simulink model "Tricopter_Controlled_development"  (R2015a)
settings: Solver=ode2  SolverMode=SingleTasking  StartTime=0.0  StopTime=inf  FixedStep=T_sim  RelTol=1e-3
values from neighbouring files (symbols this model uses):
  A_l_max_x = sqrt( (A_z_max)^2  -  g^2  )    [Run3Copter.m]
  A_l_max_y = g*tand(15)    [Run3Copter.m]
  A_x = 0.015    [SetupComplete.m]
  A_y = A_x    (= 0.015)    [SetupComplete.m]
  A_z = 0.16    [SetupComplete.m]
  A_z_max = Max_Thrust*3/m    [Run3Copter.m]
  Alt_0 = input(' Give the initial altitude (m): ')    [Run3Copter.m]
  C_x = 1.2    [SetupComplete.m]
  C_y = C_x    (= 1.2)    [SetupComplete.m]
  C_z = 2.2    [SetupComplete.m]
  CG_0 = [0,0,0.02]'    [SetupComplete.m]
  epsilon = 0.01    [Run3Copter.m]
  eta_23 = deg2rad(-1.3)    [Run3Copter.m]
  g = 9.81    [SetupComplete.m]
  h = 0.08    [SetupComplete.m]
  h_M = 0.064    [SetupComplete.m]
  I_BAC_0 = [ Ix,0,Ixz;0,Iy,0;Ixz,0,Iz]    [SetupComplete.m]
  Initial_Omegas = Omega_hover    [Run3Copter.m]
  Initial_Torques = Torque_hover    [Run3Copter.m]
  Ix = 0.103    [SetupComplete.m]
  Iy = 0.147    [SetupComplete.m]
  Iz = 0.237    [SetupComplete.m]
  l = 0.345    [SetupComplete.m]
  l_arm = 0.264    [SetupComplete.m]
  latitude = 52.071118    [Run3Copter.m]
  longitude = -0.627404    [Run3Copter.m]
  m = 3.51    [SetupComplete.m]
  m_0 = 2.61    [SetupComplete.m]
  m_M = 0.300    (= 0.3)    [SetupComplete.m]
  rho = 1.15    [SetupComplete.m]
  Rotation_sign = [ 1,-1,-1]    [SetupComplete.m]
  T_ctrl = 0.02    [Run3Copter.m]
  T_sim = 0.01    [Run3Copter.m]
  throtle_1 = 0*0.745    (= 0)    [Run3Copter.m]
  throtle_23 = throtle_1/cos(eta_23)    [Run3Copter.m]
  v_i0 = sqrt( 1/3*m*g/(2*rho*pi*R^2)  )    [SetupComplete.m]
undefined symbols (not defined in the file or in its folder): DOWN_0, EAST_0, Newton, NORTH_0, P_0, Q_0, R_0, Raphson, U_0, V_0, W_0
libraries: Adaptive_FaultTolerantControl x30, XXCopter_Control x23, simulink_extras x17, XXCopter x5, simulink x2, qcatlib x1, XXCopter_C x1
(part 4 of 4)

== matlab function Tricopter_Controlled_development/Parameters estimation/MATLAB Function ==
  data: T_yaw output; yaw input
function T_yaw = Yaw_rotate(yaw)


T_yaw=[cos(yaw),    sin(yaw),   0;
        -sin(yaw),  cos(yaw),   0;
        0,      0,              1];

== matlab function Tricopter_Controlled_development/3 Copter Complete/Ground  model/Ground model logic and Forces and moments ==
  data: Xe input; Vb input; q input; omega_b input; F_gr_b output; M_gr_b output; mass input; g parameter; Arm1 input; Arm2 input; Arm3 input
function [F_gr_b,M_gr_b]   = Gorund_Forces_and_Mom( Xe,Vb,q,omega_b,mass, g, Arm1,Arm2,Arm3)

F_gr_b=zeros(3,1);
M_gr_b=zeros(3,1);


% Arm 1
Prod=HamiltonProduct([q(1);q(2);q(3);q(4)],HamiltonProduct([0;Arm1],[q(1);-q(2);-q(3);-q(4)]) ); % q . Arm .q*: From body to earth axes
h_arm1 = Xe(3) + Prod(2:4);
% Arm 2
Prod=HamiltonProduct([q(1);q(2);q(3);q(4)],HamiltonProduct([0;Arm2],[q(1);-q(2);-q(3);-q(4)]) ); % q . Arm .q*: From body to earth axes
h_arm2 = Xe(3) + Prod(2:4);
% Arm 3
Prod=HamiltonProduct([q(1);q(2);q(3);q(4)],HamiltonProduct([0;Arm3],[q(1);-q(2);-q(3);-q(4)]) ); % q . Arm .q*: From body to earth axes
h_arm3 = Xe(3) + Prod(2:4);


min_h = max([Xe(3),h_arm1(3),h_arm2(3),h_arm3(3)]);
if min_h >=-0.01  &&  min_h <= 0  && Vb(3)>0
    Prod=HamiltonProduct([q(1);-q(2);-q(3);-q(4)],HamiltonProduct([0;0;0;-mass*g],[q(1);q(2);q(3);q(4)]) ); % q* . g .q: From earth to Body axes
    F_gr_b= Prod(2:4);
    %Friction forces
    F_gr_b = F_gr_b - 5*Vb;
    
elseif min_h >=-0.01  &&  min_h >0
    Prod=HamiltonProduct([q(1);-q(2);-q(3);-q(4)],HamiltonProduct([0;0;0; -5000*min_h ],[q(1);q(2);q(3);q(4)]) ); % q* . g .q: From earth to Body axes
    F_gr_b =  Prod(2:4);
    %Friction forces
    F_gr_b = F_gr_b - 250*Vb;
else
    F_gr_b=zeros(3,1);

end


% Moments
Prod=HamiltonProduct([q(1);-q(2);-q(3);-q(4)],HamiltonProduct([0;0;0;-mass*g],[q(1);q(2);q(3);q(4)]) ); % q* . g .q: From earth to Body axes
F_g = Prod(2:4);
if min_h >=-0.01
    if h_arm1(3)>max(h_arm2(3),h_arm3(3))+0.01
        M_gr_b=cross(Arm1,F_g);
    elseif h_arm1(3)<max(h_arm2(3),h_arm3(3))-0.01  && h_arm2(3)>h_arm3(3)+0.01
        M_gr_b=cross(Arm2,F_g);
    elseif h_arm1(3)<max(h_arm2(3),h_arm3(3))-0.01  && h_arm3(3)>h_arm2(3)+0.01
        M_gr_b=cross(Arm3,F_g);
    elseif h_arm1(3)<max(h_arm2(3),h_arm3(3))-0.01  && abs( h_arm3(3)-h_arm2(3) )<=0.01
        M_gr_b=cross( sum([Arm2,Arm3],2)/2,F_g);
        
    else
        M_gr_b=zeros(3,1);
    end
    M_gr_b = M_gr_b -10*omega_b;
else
    M_gr_b=zeros(3,1);
end
end

== matlab function Tricopter_Controlled_development/TriCopter FCS development/Inner Controller/PI Controller/MATLAB Function ==
  data: ang_dot input size=[3,1]; Omega output; euler_ang input size=[3,1]
function Omega = Euler_dot_2_omega(ang_dot,euler_ang)

phi = euler_ang(1);
theta = euler_ang(2);
psi = euler_ang(3);


A = [1          0               -sin(theta)         ;
     0          cos(phi)        sin(phi)*cos(theta) ;
     0          -sin(phi)       cos(phi)*cos(theta)];

Omega = A*ang_dot ;

== matlab function Tricopter_Controlled_development/TriCopter FCS development/Inner Controller/PI Controller Quaternions/Attitude Controller/Build Pseudo_theta ==
  data: q input; Pseudo_theta output
function Pseudo_theta    = F_Pseudo_theta( q)


%% Actitud en Angulos de Euler y sus derivadas.
Pseudo_theta=0;
Pseudo_theta = ( 2*q(2)*q(4)-2*q(1)*q(3) ); %  pseudo-theta




end

== matlab function Tricopter_Controlled_development/TriCopter FCS development/Inner Controller/PI Controller Quaternions/Attitude Controller/Build Pseudo_theta1 ==
  data: q input; Pseudo_theta output
function Pseudo_theta    = F_Pseudo_theta( q)


%% Actitud en Angulos de Euler y sus derivadas.
Pseudo_theta=0;
Pseudo_theta = ( 2*q(2)*q(4)-2*q(1)*q(3) ); %  pseudo-theta




end

== matlab function Tricopter_Controlled_development/TriCopter FCS development/Inner Controller/PI Controller Quaternions/Attitude Controller/Retrieve quaternion ==
  data: Pseudoeuler_dot input; q input; qdot output
function qdot = quat_from_Pseudoeuler(Pseudoeuler_dot, q)


%%
A = [   2/(1+( (2*q(3)*q(4)+2*q(1)*q(2))/(2*q(1)^2+2*q(4)^2-1)  )^2)*[ -(2*q(1)^2*q(2)+ 4*q(1)*q(3)*q(4)-2*q(2)*q(4)^2+q(2))  ,  q(1)*(2*q(1)^2+2*q(4)^2-1)  ,  q(4)*(2*q(1)^2+2*q(4)^2-1)  ,  -(-2*q(1)^2*q(3) +4*q(1)*q(2)*q(4)+2*q(3)*q(4)^2+q(3) ) ].* 1/(2*q(1)^2+2*q(4)^2-1)^2;...
        2*[-q(3),q(4),-q(1),q(2)];...
        2/(1+( (2*q(2)*q(3)+2*q(1)*q(4))/(2*q(1)^2+2*q(2)^2-1)  )^2)*[  -(2*q(1)^2*q(4)+4*q(1)*q(2)*q(3)-2*q(2)^2*q(4)+q(4)  ) , 1/2*(q(3)*(4*q(1)^2-4*q(2)^2-2)-8*q(1)*q(2)*q(4) )  ,  q(2)*(2*q(1)^2+2*q(2)^2-1)  , q(1)*(2*q(1)^2+2*q(2)^2-1) ].*  1/(2*q(1)^2+2*q(2)^2-1)^2 ;...
        2*[q(1),q(2),q(3),q(4)]];

qdot = pinv(A)*[Pseudoeuler_dot;0];

end

== matlab function Tricopter_Controlled_development/TriCopter FCS development/Inner Controller/PI Controller Quaternions/Get Quaternion from des euler ==
  data: phi input; q output; theta input; psi input
function q =QuaternionfromEuler(phi,theta,psi)

q=[ cos(psi/2)*cos(theta/2)*cos(phi/2)+ sin(psi/2)*sin(theta/2)*sin(phi/2) ;
      cos(psi/2)*cos(theta/2)*sin(phi/2)- sin(psi/2)*sin(theta/2)*cos(phi/2) ;
       cos(psi/2)*sin(theta/2)*cos(phi/2)+ sin(psi/2)*cos(theta/2)*sin(phi/2)   ;
        sin(psi/2)*cos(theta/2)*cos(phi/2)- cos(psi/2)*sin(theta/2)*sin(phi/2)      ]; % Esto nos da q !!!
end

== matlab function Tricopter_Controlled_development/TriCopter FCS development/Inner Controller/PI Controller Quaternions/Limits in Ang accel/Limis eval ==
  data: Ang_Accel input size=[3,1]; Limit_up output; euler_ang input size=[3,1]; Limit_down output; l parameter; m parameter; g parameter; A_l_max_x parameter; Ix parameter; Iy parameter; Iz parameter
function [Limit_up,Limit_down]= Max_ang_accels(Ang_Accel,euler_ang,l,m,g,A_l_max_x,Ix,Iy,Iz)

Limit_up=Ang_Accel;
Limit_down=Ang_Accel;

Limit_up(1) = max(   abs( (2*m*g/3*sqrt(3)/2*l  )/Ix*cos(euler_ang(1))   ), abs(  2/3*A_l_max_x*sqrt(3)/2*l/Ix*sin(euler_ang(2)) ) )* 0.5 ;
Limit_down(1) = -Limit_up(1) ;

Limit_up(2) = max(  (l*m*g*2/3-l/2*m*g/3)/Iy*cos(euler_ang(2)) , (2*l*A_l_max_x)/Iy*sin(euler_ang(2)) )* 0.5 ;
Limit_down(2) = - max( (l/2*m*g)/Iy*cos(euler_ang(2))  , (2*l*A_l_max_x)/Iy*sin(euler_ang(2)) )* 0.5 ;


Limit_up(3) = max(  abs(  A_l_max_x*l/Iz*cos(euler_ang(1))*cos(euler_ang(2)) ) , abs(  (2*m*g/3*sqrt(3)/2*l  )/Iz*sin(euler_ang(2)) )  )* 0.5 ;
Limit_down(3) = -Limit_up(1) ;

== matlab function Tricopter_Controlled_development/TriCopter FCS development/Inner Controller/PI Controller Quaternions/MATLAB Function ==
  data: omega_b input size=[3,1]; Euler_dot output; Euler input size=[3,1]
function Euler_dot = omega2Euler_dot(omega_b,Euler)

phi = Euler(1);
theta = Euler(2);
psi = Euler(3);


A = [1          0               -sin(theta)         ;
     0          cos(phi)        sin(phi)*cos(theta) ;
     0          -sin(phi)       cos(phi)*cos(theta)];

Euler_dot = A'*omega_b ;

== matlab function Tricopter_Controlled_development/TriCopter FCS development/Inner Controller/PI Controller Quaternions/Quaternion_dot ==
  data: omega_b output; q_dot input; q input
function omega_b = Quaternion_dot(q_dot,q)

% omega_b = 2.q'*q_dot
out = 2*HamiltonProduct([q(1);- q(2:4)],q_dot);

omega_b = out(2:4);

== matlab function Tricopter_Controlled_development/TriCopter FCS development/NDI/3Copter_4_NDI&CA/Get gradient ==
  data: epsilon input; CA_Grad output; Perturb_evaluations input
function CA_Grad  = Get_gradient(epsilon,Perturb_evaluations)

CA_Grad = zeros(6,9);

for i=1:9
    CA_Grad(:,i)= ( Perturb_evaluations(:,2*i)-Perturb_evaluations(:,2*i-1)  )./(epsilon);
end

%% 4 DOF
% CA_Grad(:,3)=zeros(6,1);
% CA_Grad(:,5:6)=zeros(6,2);
% CA_Grad(:,8:9)=zeros(6,2);
% 

%% Just diff throtle
% CA_Grad(3:5,2:3)=zeros(3,2);
% CA_Grad(3:5,5:6)=zeros(3,2);
% CA_Grad(3:5,8:9)=zeros(3,2);


end

== matlab function Tricopter_Controlled_development/TriCopter FCS development/NDI/3Copter_4_NDI&CA/Mass Properties/Arm Inertia ==
  data: T1_FAFb input; T2_FAFb input; T3_FAFb input; I_M output; l parameter; h_M parameter; m_M parameter; r1_M output; r2_M output; r3_M output
function [I_M,r1_M,r2_M,r3_M]  = Motor_steiner(T1_FAFb,T2_FAFb,T3_FAFb, l, h_M, m_M)


r1_M=[l;0;0]+T1_FAFb*[0;0;-h_M];
r2_M=[-1/2*l;sqrt(3)/2*l;0]+T2_FAFb*[0;0;-h_M];
r3_M=[-1/2*l;-sqrt(3)/2*l;0]+T3_FAFb*[0;0;-h_M];


I_M1 = m_M*[ r1_M(2)^2+r1_M(3)^2,r1_M(1)*r1_M(2),r1_M(1)*r1_M(3);...
            r1_M(1)*r1_M(2), r1_M(1)^2+r1_M(3)^2, r1_M(2)*r1_M(3);...
            r1_M(1)*r1_M(3),r1_M(2)*r1_M(3), r1_M(1)^2+r1_M(2)^2];
I_M2 = m_M*[ r2_M(2)^2+r2_M(3)^2,r2_M(1)*r2_M(2),r2_M(1)*r2_M(3);...
            r2_M(1)*r2_M(2), r2_M(1)^2+r2_M(3)^2, r2_M(2)*r2_M(3);...
            r2_M(1)*r2_M(3),r2_M(2)*r2_M(3), r2_M(1)^2+r2_M(2)^2];
I_M3 = m_M*[ r3_M(2)^2+r3_M(3)^2,r3_M(1)*r3_M(2),r3_M(1)*r3_M(3);...
            r3_M(1)*r3_M(2), r3_M(1)^2+r3_M(3)^2, r3_M(2)*r3_M(3);...
            r3_M(1)*r3_M(3),r3_M(2)*r3_M(3), r3_M(1)^2+r3_M(2)^2];

I_M = I_M1+I_M2+I_M3;

== matlab function Tricopter_Controlled_development/TriCopter FCS development/NDI/3Copter_4_NDI&CA/Perturbations ==
  data: epsilon input; Ctrl_input input; Pert_Ctrl output
function Pert_Ctrl  = Perturbate_input(epsilon, Ctrl_input)
% The control input has a dimension of 9
% The gradient is computed with 2 evaluations, so the output vector has
% 2*9*9 variables

Pert_Ctrl=zeros(2*9*9,1);

for i=1:9
    % Left
    tmp=Ctrl_input;
    tmp(i)=tmp(i)-epsilon;
    Pert_Ctrl( 1+2*(i-1)*9:(2*i-1)*9 ) = tmp;
    % Right
    tmp=Ctrl_input;
    tmp(i)=tmp(i)+epsilon;
    Pert_Ctrl( 1+(2*i-1)*9 :2*i*9 ) = tmp;
end






end

== matlab function Tricopter_Controlled_development/TriCopter FCS development/Outer Controller/Overactuated P Controller/MATLAB Function ==
  data: T_yaw output; yaw input
function T_yaw = Yaw_rotate(yaw)


T_yaw=[cos(yaw),    sin(yaw),   0;
        -sin(yaw),  cos(yaw),   0;
        0,      0,              1];

== matlab function Tricopter_Controlled_development/TriCopter FCS development/Outer Controller/Underactuated P Controller/Yaw rotate ==
  data: Acc_e input; Acc_yaw output; yaw input
function Acc_yaw = Yaw_rotate(Acc_e,yaw)


T=[cos(yaw),sin(yaw),0;
    -sin(yaw),cos(yaw),0;
    0,0,1];

Acc_yaw=T*Acc_e;
